simulink model "mainmodel"  (R2020a)
settings: Solver=VariableStepAuto  StartTime=0.0  StopTime=10.0  RelTol=1e-3
settings Model: Creator=Bhanu  LastModifiedBy=Bhanu

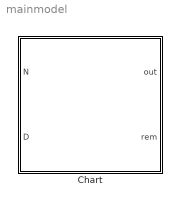
== system mainmodel ==
  Chart : Stateflow chart  TreatAsAtomicUnit=on

== stateflow chart mainmodel/Chart ==
  settings: stateMachineType=MEALY_MACHINE
  state zero_cents
  state five_cents
  (default) -> zero_cents
  zero_cents -> zero_cents [order 3] : [D == 1]/{out = 0}
  five_cents -> five_cents [order 3] : [N == 0 || D == 0]/{out = 0}
  zero_cents -> five_cents [order 1] : [N == 1]/{out = 0}
  zero_cents -> zero_cents [order 2] : [N == 0 && D == 0]/{out = 0}
  five_cents -> zero_cents [order 1] : [N == 1]/{out = 1}
  five_cents -> zero_cents [order 2] : [D == 1]/{out = 1 && rem == 5}
  data: N input; D input; out output; rem output =0
